simulink model "id_openloop"  (R2017a)
settings: Solver=ode45  StartTime=0.0  StopTime=5000  RelTol=1e-3  EnableMultiTasking=on
values from neighbouring files (symbols this model uses):
  a = 0    [OE_Ident.m]    (also in fast.m = zeros(DMAX-DMIN+1,1); golden.m = h)
settings Model: ExtModeTrigMode=oneshot  ExtModeArmWhenConnect=off  Creator=The MathWorks, Inc.  LastModifiedBy=Geethanzali
settings DataIOCC: SaveFormat=Array
settings OptimizationCC: BooleanDataType=off  InitFltsAndDblsToZero=on  LifeSpan=inf
settings DebuggingCC: SaveWithParameterizedLinksMsg=none  UnderspecifiedInitializationDetection=Classic  MergeDetectMultiDrivingBlocksExec=none  SignalResolutionControl=TryResolveAllWithWarning  MultiTaskDSMMsg=warning  MultiTaskCondExecSysMsg=none  IntegerOverflowMsg=none  FcnCallInpInsideContextMsg=warning  SFUnexpectedBacktrackingDiag=warning  SFNoUnconditionalDefaultTransitionDiag=warning  SFExecutionAtInitializationDiag=none  IntegerSaturationMsg=none
settings HardwareCC: ProdBitPerPointer=32  ProdBitPerSizeT=32  ProdBitPerPtrDiffT=32  ProdLargestAtomicFloat=None  ProdIntDivRoundTo=Undefined  ProdEndianess=Unspecified  ProdWordSize=32  ProdHWDeviceType=32-bit Generic  TargetUnknown=on
settings ModelReferenceCC: PropagateSignalLabelsOutOfModel=off
settings GRTTargetCC: TargetFcnLib=ansi_tfl_tmw.mat  TargetLangStandard=C89/C90 (ANSI)  CombineOutputUpdateFcns=off  GRTInterface=on
settings ConfigComp: CovMetricSettings=dw  CovHtmlReporting=on  CovSaveCumulativeToWorkspaceVar=on  CovSaveSingleToWorkspaceVar=on  CovExternalEMLEnable=off

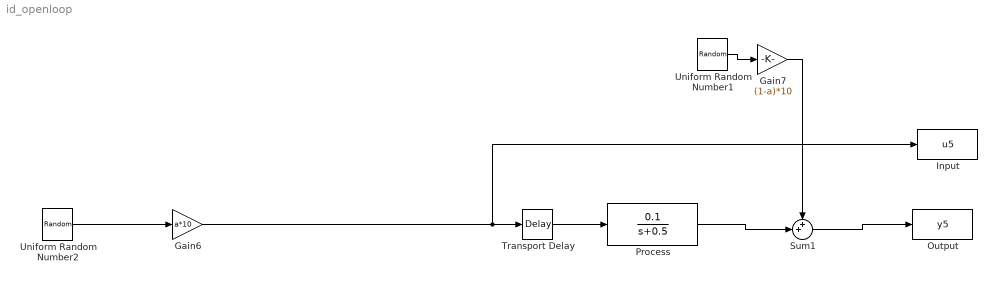
== system id_openloop ==
  Gain6 : Gain  Gain=a*10  SaturateOnIntegerOverflow=on  OutDataTypeStr=Inherit: Same as input  ParamDataTypeStr=Inherit: Same as input
  Gain7 : Gain  Gain=(1-a)*10  SaturateOnIntegerOverflow=on  OutDataTypeStr=Inherit: Same as input  ParamDataTypeStr=Inherit: Same as input
  Input : ToWorkspace  VariableName=u5  SampleTime=0.5
  Output : ToWorkspace  VariableName=y5  SampleTime=0.5
  "Process " : TransferFcn  Numerator=0.1  Denominator=[1 0.5]
  Sum1 : Sum  Inputs=++|
  Transport Delay : TransportDelay  DelayTime=1.57
  Uniform Random Number1 : UniformRandomNumber  Minimum=0  Maximum=10  SampleTime=20
  Uniform Random Number2 : UniformRandomNumber  Minimum=0  Maximum=10  SampleTime=20
  wires:
  Uniform Random Number1/1 -> Gain7/1
  Gain6/1 -> Input/1, Transport Delay/1
  Transport Delay/1 -> "Process "/1
  "Process "/1 -> Sum1/2
  Sum1/1 -> Output/1
  Gain7/1 -> Sum1/1
  Uniform Random Number2/1 -> Gain6/1
